simulink model "VSC_GF_2bus_nonlinear"  (R2021b)
settings: Solver=ode45  StartTime=0.0  StopTime=Tsim  FixedStep=10e-6  RelTol=1e-6  EnableMultiTasking=on
values from neighbouring files (symbols this model uses):
  angle_g1_fnl = 0.0    (= 0)    [params_pu.m]
  angle_g1_init = 0.0    (= 0)    [params_pu.m]
  Cac_n1 = 0.15/wb_n1    (= 0.000477464829276)    [params_pu.m]
  k_droop_u_n1 = (0.02/0.3)*(sqrt(2)/sqrt(3))    [params_pu.m]
  ki_pll1 = kp_pll1/tau_pll_n1    [params_pu.m]
  ki_vac_n1 = 42.05*(Vb_n1/Ib_n1)    (= 7.28000181818)    [params_pu.m]
  kp_pll1 = xi_pll_n1*2*omega_pll_n1/(sqrt(2)/sqrt(3))    [params_pu.m]
  kp_vac_n1 = 4.789*(Vb_n1/Ib_n1)    (= 0.829106509091)    [params_pu.m]
  Lc_n1 = 0.15/wb_n1    (= 0.000477464829276)    [params_pu.m]
  Lg_n1 = Xg_n1/wb_n1    [params_pu.m]
  Lg_n2 = imag(Zg_n2)/wb_n1    [params_pu.m]
  magnitud_delay = 1e-5    (= 1e-05)    [params_pu.m]
  P_ref_n1 = 0.5    [params_pu.m]
  plots_step = 10e-6    (= 1e-05)    [params_pu.m]
  Q_ref_n1 = 0.1    [params_pu.m]
  Rac_n1 = 1/(3*10*wb_n1*Cac_n1)    (= 0.222222222222)    [params_pu.m]
  Rg_n1 = Rg_n1/Zb_n1    [params_pu.m]
  Rg_n2 = real(Zg_n2)    [params_pu.m]
  Rseries_n1 = 5e-4/Zb_n1    (= 0.00288804872926)    [params_pu.m]
  T_stp = Tsim/2    (= 2)    [params_pu.m]
  tau_droop_f = 1/50    (= 0.02)    [params_pu.m]
  tau_droop_u = 1/50    (= 0.02)    [params_pu.m]
  tau_ig = 0.1e-3    (= 0.0001)    [params_pu.m]
  tau_u = 0.1e-3    (= 0.0001)    [params_pu.m]
  Vb_dc_n1 = 2e3    (= 2000)    [params_pu.m]
  Vb_n1 = 0.69e3    (= 690)    [params_pu.m]
  Vdcref_n1 = Vb_dc_n1    (= 2000)    [params_pu.m]
  Vpeak_g1_fnl = 0.98*(sqrt(2)/sqrt(3))    [params_pu.m]
  Vpeak_g1_init = 1*(sqrt(2)/sqrt(3))    [params_pu.m]
  Vpeak_n1 = Vb_n1/sqrt(3)*sqrt(2)    [params_pu.m]
  wb_n1 = 2*pi*fb_n1    (= 314.159265359)    [params_pu.m]
undefined symbols (not defined in the file or in its folder): Cac, DRload, Ib_vsc, is_dc0, is_qc0, k_droop_f, ki_s, ki_vac, kp_s, kp_vac, Lc, Lf, Ltr, P, Rac, Rc, Rtr, Sb, T_load, tstep, u_dc0, u_q0, u_qc0, Vb_vsc, vc_dc0, vc_qc0, wb, Zb
libraries: spsSeriesRLCBranchLib x42, spsParallelRLCBranchLib x21, spsControlledVoltageSourceLib x14, spsCurrentMeasurementLib x14, spsGroundLib x10, slpidlib x9, spsVoltageMeasurementLib x6, spsThreePhaseVIMeasurementLib x2, spsPower3phInstantaneousLib x2, spsThreePhaseBreakerLib x2, spsControlledCurrentSourceLib x2, eeTransforms x1
(part 3 of 3)

== system VSC_GF_2bus_nonlinear/ParkTransform5 ==
  ABC vector : Inport
  angle : Inport  Port=2
  Constant1 : Constant  Value=1/2
  Constant2 : Constant  Value=1/2
  Constant3 : Constant  Value=2*pi/3
  Constant4 : Constant  Value=2*pi/3
  Constant5 : Constant  Value=1/2
  Gain : Gain  Gain=2/3
  Matrix Concatenate : Concatenate  NumInputs=3  Mode=Multidimensional array  ConcatenateDimension=2
  Mux1 : Mux  Inputs=3
  Mux2 : Mux  Inputs=3
  Mux3 : Mux  Inputs=3
  Product : Product  Multiplication=Matrix(*)  RndMeth=Zero
  Sum : Sum  Inputs=|+-
  Sum1 : Sum  Inputs=|++
  Trigonometric Function1 : Trigonometry  Operator=cos
  Trigonometric Function2 : Trigonometry  Operator=cos
  Trigonometric Function3 : Trigonometry
  Trigonometric Function4 : Trigonometry
  Trigonometric Function5 : Trigonometry  Operator=cos
  Trigonometric Function6 : Trigonometry
  Matrix : Outport
  wires:
  Mux3/1 -> Matrix Concatenate/3
  Mux2/1 -> Matrix Concatenate/1
  Mux1/1 -> Matrix Concatenate/2
  Sum1/1 -> Trigonometric Function5/1, Trigonometric Function6/1
  Constant5/1 -> Mux3/3
  Trigonometric Function5/1 -> Mux3/1
  Trigonometric Function6/1 -> Mux3/2
  Constant1/1 -> Mux2/3
  Trigonometric Function1/1 -> Mux2/1
  Trigonometric Function4/1 -> Mux2/2
  Sum/1 -> Trigonometric Function2/1, Trigonometric Function3/1
  Constant2/1 -> Mux1/3
  Trigonometric Function2/1 -> Mux1/1
  Trigonometric Function3/1 -> Mux1/2
  angle/1 -> Sum/1, Sum1/1, Trigonometric Function1/1, Trigonometric Function4/1
  Constant3/1 -> Sum1/2
  Constant4/1 -> Sum/2
  Gain/1 -> Product/1
  Product/1 -> Matrix/1
  ABC vector/1 -> Product/2
  Matrix Concatenate/1 -> Gain/1

== system VSC_GF_2bus_nonlinear/ParkTransform6 ==
  ABC vector : Inport
  angle : Inport  Port=2
  Constant1 : Constant  Value=1/2
  Constant2 : Constant  Value=1/2
  Constant3 : Constant  Value=2*pi/3
  Constant4 : Constant  Value=2*pi/3
  Constant5 : Constant  Value=1/2
  Gain : Gain  Gain=2/3
  Matrix Concatenate : Concatenate  NumInputs=3  Mode=Multidimensional array  ConcatenateDimension=2
  Mux1 : Mux  Inputs=3
  Mux2 : Mux  Inputs=3
  Mux3 : Mux  Inputs=3
  Product : Product  Multiplication=Matrix(*)  RndMeth=Zero
  Sum : Sum  Inputs=|+-
  Sum1 : Sum  Inputs=|++
  Trigonometric Function1 : Trigonometry  Operator=cos
  Trigonometric Function2 : Trigonometry  Operator=cos
  Trigonometric Function3 : Trigonometry
  Trigonometric Function4 : Trigonometry
  Trigonometric Function5 : Trigonometry  Operator=cos
  Trigonometric Function6 : Trigonometry
  Matrix : Outport
  wires:
  Mux3/1 -> Matrix Concatenate/3
  Mux2/1 -> Matrix Concatenate/1
  Mux1/1 -> Matrix Concatenate/2
  Sum1/1 -> Trigonometric Function5/1, Trigonometric Function6/1
  Constant5/1 -> Mux3/3
  Trigonometric Function5/1 -> Mux3/1
  Trigonometric Function6/1 -> Mux3/2
  Constant1/1 -> Mux2/3
  Trigonometric Function1/1 -> Mux2/1
  Trigonometric Function4/1 -> Mux2/2
  Sum/1 -> Trigonometric Function2/1, Trigonometric Function3/1
  Constant2/1 -> Mux1/3
  Trigonometric Function2/1 -> Mux1/1
  Trigonometric Function3/1 -> Mux1/2
  angle/1 -> Sum/1, Sum1/1, Trigonometric Function1/1, Trigonometric Function4/1
  Constant3/1 -> Sum1/2
  Constant4/1 -> Sum/2
  Gain/1 -> Product/1
  Product/1 -> Matrix/1
  ABC vector/1 -> Product/2
  Matrix Concatenate/1 -> Gain/1

== system VSC_GF_2bus_nonlinear/ParkTransform8 ==
  ABC vector : Inport
  angle : Inport  Port=2
  Constant1 : Constant  Value=1/2
  Constant2 : Constant  Value=1/2
  Constant3 : Constant  Value=2*pi/3
  Constant4 : Constant  Value=2*pi/3
  Constant5 : Constant  Value=1/2
  Gain : Gain  Gain=2/3
  Matrix Concatenate : Concatenate  NumInputs=3  Mode=Multidimensional array  ConcatenateDimension=2
  Mux1 : Mux  Inputs=3
  Mux2 : Mux  Inputs=3
  Mux3 : Mux  Inputs=3
  Product : Product  Multiplication=Matrix(*)  RndMeth=Zero
  Sum : Sum  Inputs=|+-
  Sum1 : Sum  Inputs=|++
  Trigonometric Function1 : Trigonometry  Operator=cos
  Trigonometric Function2 : Trigonometry  Operator=cos
  Trigonometric Function3 : Trigonometry
  Trigonometric Function4 : Trigonometry
  Trigonometric Function5 : Trigonometry  Operator=cos
  Trigonometric Function6 : Trigonometry
  Matrix : Outport
  wires:
  Matrix Concatenate/1 -> Gain/1
  ABC vector/1 -> Product/2
  Product/1 -> Matrix/1
  Gain/1 -> Product/1
  Constant4/1 -> Sum/2
  Constant3/1 -> Sum1/2
  angle/1 -> Trigonometric Function4/1, Trigonometric Function1/1, Sum1/1, Sum/1
  Trigonometric Function3/1 -> Mux1/2
  Trigonometric Function2/1 -> Mux1/1
  Constant2/1 -> Mux1/3
  Sum/1 -> Trigonometric Function3/1, Trigonometric Function2/1
  Trigonometric Function4/1 -> Mux2/2
  Trigonometric Function1/1 -> Mux2/1
  Constant1/1 -> Mux2/3
  Trigonometric Function6/1 -> Mux3/2
  Trigonometric Function5/1 -> Mux3/1
  Constant5/1 -> Mux3/3
  Sum1/1 -> Trigonometric Function6/1, Trigonometric Function5/1
  Mux1/1 -> Matrix Concatenate/2
  Mux2/1 -> Matrix Concatenate/1
  Mux3/1 -> Matrix Concatenate/3

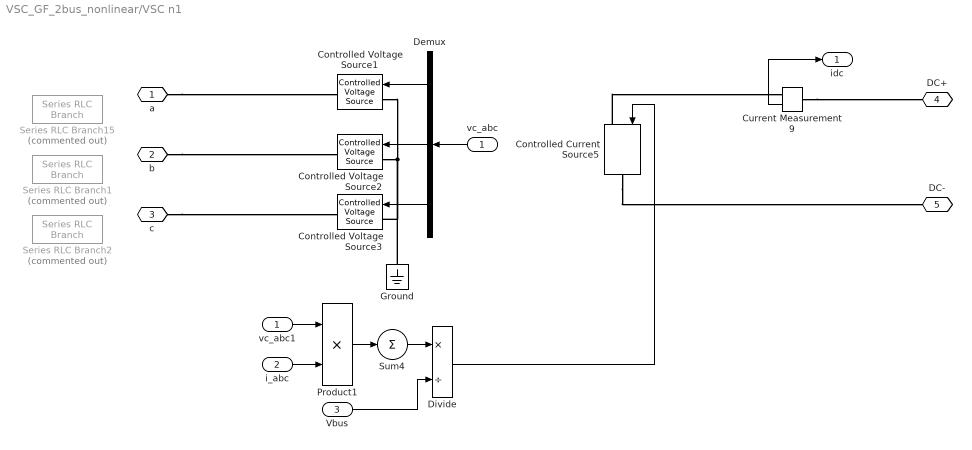
== system VSC_GF_2bus_nonlinear/VSC n1 ==
  vc_abc : Inport
  i_abc : Inport  Port=2
  Vbus : Inport  Port=3
  Controlled Current Source5 : spsControlledCurrentSourceLib/Controlled Current Source  Initialize=on  Source_Type=DC  Amplitude=0  Phase=0  Frequency=0  Measurements=None
  Controlled Voltage Source1 : spsControlledVoltageSourceLib/Controlled Voltage Source  Initialize=off  Source_Type=AC  Amplitude=0  Phase=0  Frequency=0  Measurements=None
  Controlled Voltage Source2 : spsControlledVoltageSourceLib/Controlled Voltage Source  Initialize=off  Source_Type=AC  Amplitude=0  Phase=0  Frequency=0  Measurements=None
  Controlled Voltage Source3 : spsControlledVoltageSourceLib/Controlled Voltage Source  Initialize=off  Source_Type=AC  Amplitude=0  Phase=0  Frequency=0  Measurements=None
  Current Measurement9 : spsCurrentMeasurementLib/Current Measurement  PhasorSimulation=off  OutputType=Complex  PSBequivalent=0
  Demux : Demux  Outputs=3
  Divide : Product  Inputs=*/
  Ground : spsGroundLib/Ground  LConnTagsString=a
  Product1 : Product  InputSameDT=on  SaturateOnIntegerOverflow=on  OutDataTypeStr=Inherit: Same as first input
  Series RLC Branch1 : spsSeriesRLCBranchLib/Series RLC Branch  Commented=on  LConnTagsString=__new0  RConnTagsString=__new0  BranchType=R  Resistance=Rseries_n1  Inductance=Lc_n1  SetiL0=off  InitialCurrent=0  Capacitance=0  Setx0=off  InitialVoltage=0  Measurements=None
  Series RLC Branch15 : spsSeriesRLCBranchLib/Series RLC Branch  Commented=on  LConnTagsString=__new0  RConnTagsString=__new0  BranchType=R  Resistance=Rseries_n1  Inductance=Lc_n1  SetiL0=off  InitialCurrent=0  Capacitance=0  Setx0=off  InitialVoltage=0  Measurements=None
  Series RLC Branch2 : spsSeriesRLCBranchLib/Series RLC Branch  Commented=on  LConnTagsString=__new0  RConnTagsString=__new0  BranchType=R  Resistance=Rseries_n1  Inductance=Lc_n1  SetiL0=off  InitialCurrent=0  Capacitance=0  Setx0=off  InitialVoltage=0  Measurements=None
  Sum4 : Sum  Inputs=1  InputSameDT=on  SaturateOnIntegerOverflow=on  OutDataTypeStr=Inherit: Same as first input
  vc_abc1 : InportShadow
  a : PMIOPort  Side=Left
  b : PMIOPort  Port=2  Side=Left
  c : PMIOPort  Port=3  Side=Left
  DC+ : PMIOPort  Port=4  Side=Right
  DC- : PMIOPort  Port=5  Side=Right
  idc : Outport
  wires:
  Current Measurement9/1 -> idc/1
  Product1/1 -> Sum4/1
  Sum4/1 -> Divide/1
  Divide/1 -> Controlled Current Source5/1
  vc_abc1/1 -> Product1/1
  i_abc/1 -> Product1/2
  Demux/2 -> Controlled Voltage Source2/1
  Demux/1 -> Controlled Voltage Source1/1
  Demux/3 -> Controlled Voltage Source3/1
  vc_abc/1 -> Demux/1
  Vbus/1 -> Divide/2
  connections:
  Controlled Current Source5/RConn1 -- DC-/RConn1
  Controlled Current Source5/LConn1 -- Current Measurement9/RConn1
  Current Measurement9/LConn1 -- DC+/RConn1
  Controlled Voltage Source1/LConn1 -- Ground/LConn1 -- Controlled Voltage Source3/LConn1 -- Controlled Voltage Source2/LConn1
  a/RConn1 -- Controlled Voltage Source1/RConn1
  b/RConn1 -- Controlled Voltage Source2/RConn1
  c/RConn1 -- Controlled Voltage Source3/RConn1

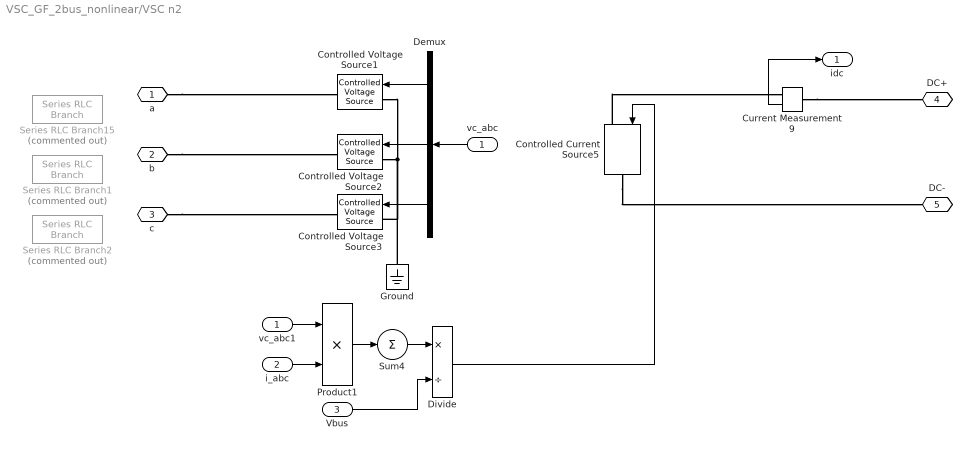
== system VSC_GF_2bus_nonlinear/VSC n2 ==
  vc_abc : Inport
  i_abc : Inport  Port=2
  Vbus : Inport  Port=3
  Controlled Current Source5 : spsControlledCurrentSourceLib/Controlled Current Source  Initialize=on  Source_Type=DC  Amplitude=0  Phase=0  Frequency=0  Measurements=None
  Controlled Voltage Source1 : spsControlledVoltageSourceLib/Controlled Voltage Source  Initialize=off  Source_Type=AC  Amplitude=0  Phase=0  Frequency=0  Measurements=None
  Controlled Voltage Source2 : spsControlledVoltageSourceLib/Controlled Voltage Source  Initialize=off  Source_Type=AC  Amplitude=0  Phase=0  Frequency=0  Measurements=None
  Controlled Voltage Source3 : spsControlledVoltageSourceLib/Controlled Voltage Source  Initialize=off  Source_Type=AC  Amplitude=0  Phase=0  Frequency=0  Measurements=None
  Current Measurement9 : spsCurrentMeasurementLib/Current Measurement  PhasorSimulation=off  OutputType=Complex  PSBequivalent=0
  Demux : Demux  Outputs=3
  Divide : Product  Inputs=*/
  Ground : spsGroundLib/Ground  LConnTagsString=a
  Product1 : Product  InputSameDT=on  SaturateOnIntegerOverflow=on  OutDataTypeStr=Inherit: Same as first input
  Series RLC Branch1 : spsSeriesRLCBranchLib/Series RLC Branch  Commented=on  LConnTagsString=__new0  RConnTagsString=__new0  BranchType=R  Resistance=Rseries_n1  Inductance=Lc_n1  SetiL0=off  InitialCurrent=0  Capacitance=0  Setx0=off  InitialVoltage=0  Measurements=None
  Series RLC Branch15 : spsSeriesRLCBranchLib/Series RLC Branch  Commented=on  LConnTagsString=__new0  RConnTagsString=__new0  BranchType=R  Resistance=Rseries_n1  Inductance=Lc_n1  SetiL0=off  InitialCurrent=0  Capacitance=0  Setx0=off  InitialVoltage=0  Measurements=None
  Series RLC Branch2 : spsSeriesRLCBranchLib/Series RLC Branch  Commented=on  LConnTagsString=__new0  RConnTagsString=__new0  BranchType=R  Resistance=Rseries_n1  Inductance=Lc_n1  SetiL0=off  InitialCurrent=0  Capacitance=0  Setx0=off  InitialVoltage=0  Measurements=None
  Sum4 : Sum  Inputs=1  InputSameDT=on  SaturateOnIntegerOverflow=on  OutDataTypeStr=Inherit: Same as first input
  vc_abc1 : InportShadow
  a : PMIOPort  Side=Left
  b : PMIOPort  Port=2  Side=Left
  c : PMIOPort  Port=3  Side=Left
  DC+ : PMIOPort  Port=4  Side=Right
  DC- : PMIOPort  Port=5  Side=Right
  idc : Outport
  wires:
  Current Measurement9/1 -> idc/1
  Product1/1 -> Sum4/1
  Sum4/1 -> Divide/1
  Divide/1 -> Controlled Current Source5/1
  vc_abc1/1 -> Product1/1
  i_abc/1 -> Product1/2
  Demux/2 -> Controlled Voltage Source2/1
  Demux/1 -> Controlled Voltage Source1/1
  Demux/3 -> Controlled Voltage Source3/1
  vc_abc/1 -> Demux/1
  Vbus/1 -> Divide/2
  connections:
  Controlled Current Source5/RConn1 -- DC-/RConn1
  Controlled Current Source5/LConn1 -- Current Measurement9/RConn1
  Current Measurement9/LConn1 -- DC+/RConn1
  Controlled Voltage Source1/LConn1 -- Ground/LConn1 -- Controlled Voltage Source3/LConn1 -- Controlled Voltage Source2/LConn1
  a/RConn1 -- Controlled Voltage Source1/RConn1
  b/RConn1 -- Controlled Voltage Source2/RConn1
  c/RConn1 -- Controlled Voltage Source3/RConn1

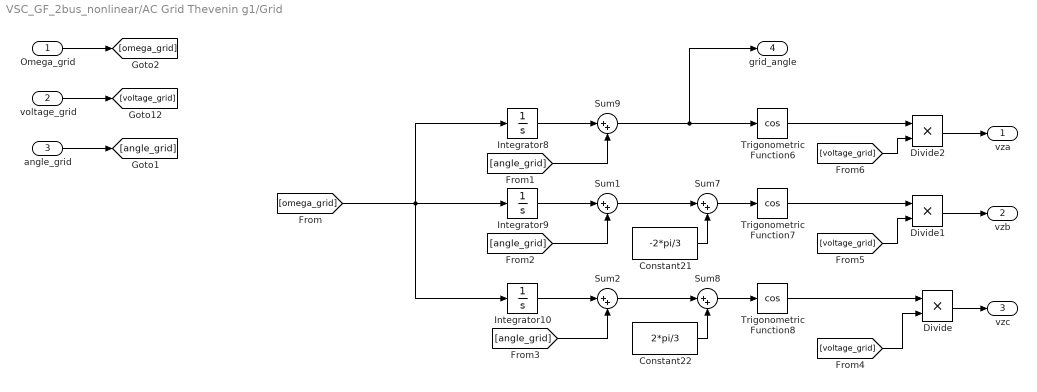
== system VSC_GF_2bus_nonlinear/AC Grid Thevenin g1/Grid ==
  Omega_grid : Inport
  voltage_grid : Inport  Port=2
  angle_grid : Inport  Port=3
  Constant21 : Constant  Value=-2*pi/3
  Constant22 : Constant  Value=2*pi/3
  Divide : Product  Inputs=**
  Divide1 : Product  Inputs=**
  Divide2 : Product  Inputs=**
  Integrator10 : Integrator
  Integrator8 : Integrator
  Integrator9 : Integrator
  Sum{1..2,7..9} (5 alike) : Sum  Inputs=|++
  Trigonometric Function6 : Trigonometry  Operator=cos
  Trigonometric Function7 : Trigonometry  Operator=cos
  Trigonometric Function8 : Trigonometry  Operator=cos
  vza : Outport  VectorParamsAs1DForOutWhenUnconnected=off
  vzb : Outport  Port=2  VectorParamsAs1DForOutWhenUnconnected=off
  vzc : Outport  Port=3  VectorParamsAs1DForOutWhenUnconnected=off
  grid_angle : Outport  Port=4  VectorParamsAs1DForOutWhenUnconnected=off
  wires:
  Trigonometric Function8/1 -> Divide/1
  Trigonometric Function7/1 -> Divide1/1
  Sum9/1 -> grid_angle/1, Trigonometric Function6/1
  Constant22/1 -> Sum8/2
  Sum2/1 -> Sum8/1
  Constant21/1 -> Sum7/2
  Integrator8/1 -> Sum9/1
  Sum7/1 -> Trigonometric Function7/1
  [angle_grid] -> Sum9/2
  Sum1/1 -> Sum7/1
  Sum8/1 -> Trigonometric Function8/1
  Trigonometric Function6/1 -> Divide2/1
  [voltage_grid] -> Divide/2
  Divide/1 -> vzc/1
  Divide1/1 -> vzb/1
  Divide2/1 -> vza/1
  Integrator9/1 -> Sum1/1
  angle_grid/1 -> [angle_grid]
  voltage_grid/1 -> [voltage_grid]
  Omega_grid/1 -> [omega_grid]
  [omega_grid] -> Integrator10/1, Integrator8/1, Integrator9/1
  [angle_grid] -> Sum1/2
  Integrator10/1 -> Sum2/1
  [angle_grid] -> Sum2/2
  [voltage_grid] -> Divide1/2
  [voltage_grid] -> Divide2/2

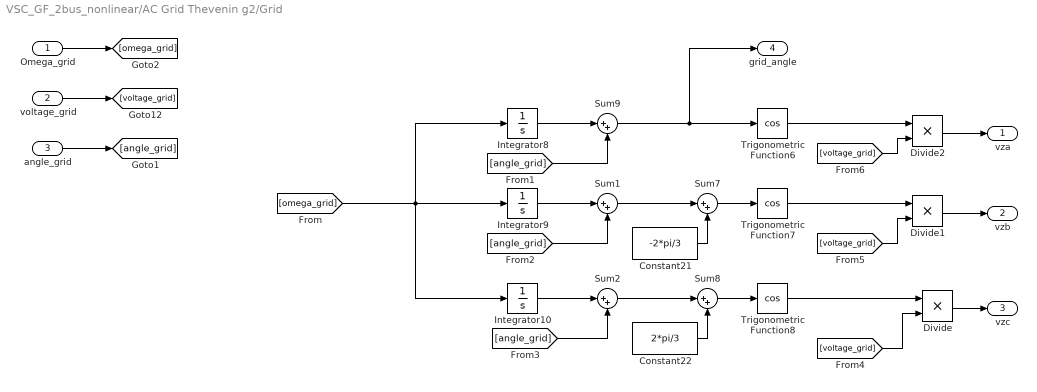
== system VSC_GF_2bus_nonlinear/AC Grid Thevenin g2/Grid ==
  Omega_grid : Inport
  voltage_grid : Inport  Port=2
  angle_grid : Inport  Port=3
  Constant21 : Constant  Value=-2*pi/3
  Constant22 : Constant  Value=2*pi/3
  Divide : Product  Inputs=**
  Divide1 : Product  Inputs=**
  Divide2 : Product  Inputs=**
  Integrator10 : Integrator
  Integrator8 : Integrator
  Integrator9 : Integrator
  Sum{1..2,7..9} (5 alike) : Sum  Inputs=|++
  Trigonometric Function6 : Trigonometry  Operator=cos
  Trigonometric Function7 : Trigonometry  Operator=cos
  Trigonometric Function8 : Trigonometry  Operator=cos
  vza : Outport  VectorParamsAs1DForOutWhenUnconnected=off
  vzb : Outport  Port=2  VectorParamsAs1DForOutWhenUnconnected=off
  vzc : Outport  Port=3  VectorParamsAs1DForOutWhenUnconnected=off
  grid_angle : Outport  Port=4  VectorParamsAs1DForOutWhenUnconnected=off
  wires:
  Trigonometric Function8/1 -> Divide/1
  Trigonometric Function7/1 -> Divide1/1
  Sum9/1 -> grid_angle/1, Trigonometric Function6/1
  Constant22/1 -> Sum8/2
  Sum2/1 -> Sum8/1
  Constant21/1 -> Sum7/2
  Integrator8/1 -> Sum9/1
  Sum7/1 -> Trigonometric Function7/1
  [angle_grid] -> Sum9/2
  Sum1/1 -> Sum7/1
  Sum8/1 -> Trigonometric Function8/1
  Trigonometric Function6/1 -> Divide2/1
  [voltage_grid] -> Divide/2
  Divide/1 -> vzc/1
  Divide1/1 -> vzb/1
  Divide2/1 -> vza/1
  Integrator9/1 -> Sum1/1
  angle_grid/1 -> [angle_grid]
  voltage_grid/1 -> [voltage_grid]
  Omega_grid/1 -> [omega_grid]
  [omega_grid] -> Integrator10/1, Integrator8/1, Integrator9/1
  [angle_grid] -> Sum1/2
  Integrator10/1 -> Sum2/1
  [angle_grid] -> Sum2/2
  [voltage_grid] -> Divide1/2
  [voltage_grid] -> Divide2/2

== system VSC_GF_2bus_nonlinear/Current regulator/ParkInverse ==
  ABC vector : Inport
  angle : Inport  Port=2
  Constant4 : Constant  Value=2*pi/3
  Constant5 : Constant  Value=2*pi/3
  Constant9 : Constant
  Matrix Concatenate2 : Concatenate  NumInputs=3  Mode=Multidimensional array  ConcatenateDimension=2
  Mux6 : Mux  Inputs=3
  Mux7 : Mux  Inputs=3
  Product : Product  Multiplication=Matrix(*)  RndMeth=Zero
  Sum : Sum  Inputs=|+-
  Sum1 : Sum  Inputs=|++
  Trigonometric Function8 : Trigonometry  Operator=cos
  Trigonometric Function9 : Trigonometry
  Matrix : Outport
  wires:
  angle/1 -> Sum1/1, Sum/1, Mux6/1
  Constant5/1 -> Sum1/2
  Constant4/1 -> Sum/2
  Product/1 -> Matrix/1
  ABC vector/1 -> Product/2
  Sum/1 -> Mux6/2
  Sum1/1 -> Mux6/3
  Constant9/1 -> Mux7/3, Mux7/1, Mux7/2
  Trigonometric Function8/1 -> Matrix Concatenate2/1
  Trigonometric Function9/1 -> Matrix Concatenate2/2
  Mux6/1 -> Trigonometric Function9/1, Trigonometric Function8/1
  Mux7/1 -> Matrix Concatenate2/3
  Matrix Concatenate2/1 -> Product/1

== system VSC_GF_2bus_nonlinear/Current regulator1/ParkInverse ==
  ABC vector : Inport
  angle : Inport  Port=2
  Constant4 : Constant  Value=2*pi/3
  Constant5 : Constant  Value=2*pi/3
  Constant9 : Constant
  Matrix Concatenate2 : Concatenate  NumInputs=3  Mode=Multidimensional array  ConcatenateDimension=2
  Mux6 : Mux  Inputs=3
  Mux7 : Mux  Inputs=3
  Product : Product  Multiplication=Matrix(*)  RndMeth=Zero
  Sum : Sum  Inputs=|+-
  Sum1 : Sum  Inputs=|++
  Trigonometric Function8 : Trigonometry  Operator=cos
  Trigonometric Function9 : Trigonometry
  Matrix : Outport
  wires:
  angle/1 -> Sum1/1, Sum/1, Mux6/1
  Constant5/1 -> Sum1/2
  Constant4/1 -> Sum/2
  Product/1 -> Matrix/1
  ABC vector/1 -> Product/2
  Sum/1 -> Mux6/2
  Sum1/1 -> Mux6/3
  Constant9/1 -> Mux7/3, Mux7/1, Mux7/2
  Trigonometric Function8/1 -> Matrix Concatenate2/1
  Trigonometric Function9/1 -> Matrix Concatenate2/2
  Mux6/1 -> Trigonometric Function9/1, Trigonometric Function8/1
  Mux7/1 -> Matrix Concatenate2/3
  Matrix Concatenate2/1 -> Product/1

== system VSC_GF_2bus_nonlinear/PLL/ParkTransform7 ==
  ABC vector : Inport
  angle : Inport  Port=2
  Constant1 : Constant  Value=1/2
  Constant2 : Constant  Value=1/2
  Constant3 : Constant  Value=2*pi/3
  Constant4 : Constant  Value=2*pi/3
  Constant5 : Constant  Value=1/2
  Gain : Gain  Gain=2/3
  Matrix Concatenate : Concatenate  NumInputs=3  Mode=Multidimensional array  ConcatenateDimension=2
  Mux1 : Mux  Inputs=3
  Mux2 : Mux  Inputs=3
  Mux3 : Mux  Inputs=3
  Product : Product  Multiplication=Matrix(*)  RndMeth=Zero
  Sum : Sum  Inputs=|+-
  Sum1 : Sum  Inputs=|++
  Trigonometric Function1 : Trigonometry  Operator=cos
  Trigonometric Function2 : Trigonometry  Operator=cos
  Trigonometric Function3 : Trigonometry
  Trigonometric Function4 : Trigonometry
  Trigonometric Function5 : Trigonometry  Operator=cos
  Trigonometric Function6 : Trigonometry
  Matrix : Outport
  wires:
  Mux3/1 -> Matrix Concatenate/3
  Mux2/1 -> Matrix Concatenate/1
  Mux1/1 -> Matrix Concatenate/2
  Sum1/1 -> Trigonometric Function5/1, Trigonometric Function6/1
  Constant5/1 -> Mux3/3
  Trigonometric Function5/1 -> Mux3/1
  Trigonometric Function6/1 -> Mux3/2
  Constant1/1 -> Mux2/3
  Trigonometric Function1/1 -> Mux2/1
  Trigonometric Function4/1 -> Mux2/2
  Sum/1 -> Trigonometric Function2/1, Trigonometric Function3/1
  Constant2/1 -> Mux1/3
  Trigonometric Function2/1 -> Mux1/1
  Trigonometric Function3/1 -> Mux1/2
  angle/1 -> Sum/1, Sum1/1, Trigonometric Function1/1, Trigonometric Function4/1
  Constant3/1 -> Sum1/2
  Constant4/1 -> Sum/2
  Gain/1 -> Product/1
  Product/1 -> Matrix/1
  ABC vector/1 -> Product/2
  Matrix Concatenate/1 -> Gain/1
